simulink model "MVC2025_sim"  (R2024b)
settings: Solver=FixedStepAuto  StartTime=0.0  StopTime=Tsim  FixedStep=Ts
InitFcn:
  | warning('off','all')
StopFcn:
  | warning('on','all')
undefined symbols (not defined in the file or in its folder): BAT, BUS, CTRLpmsm, CTRLtug, CTRLves, DiscIntNeverNeededParam, ESM, GEN, magnitude, MOT, RLgain, SM, tau0, Ts, TUG, VES
libraries: fl_lib x47, nesl_utility x35, simulink x24, slpidlib x10, ee_lib x10, sdl_lib x3, rllib x1, batteryecm_lib x1
(part 3 of 3)

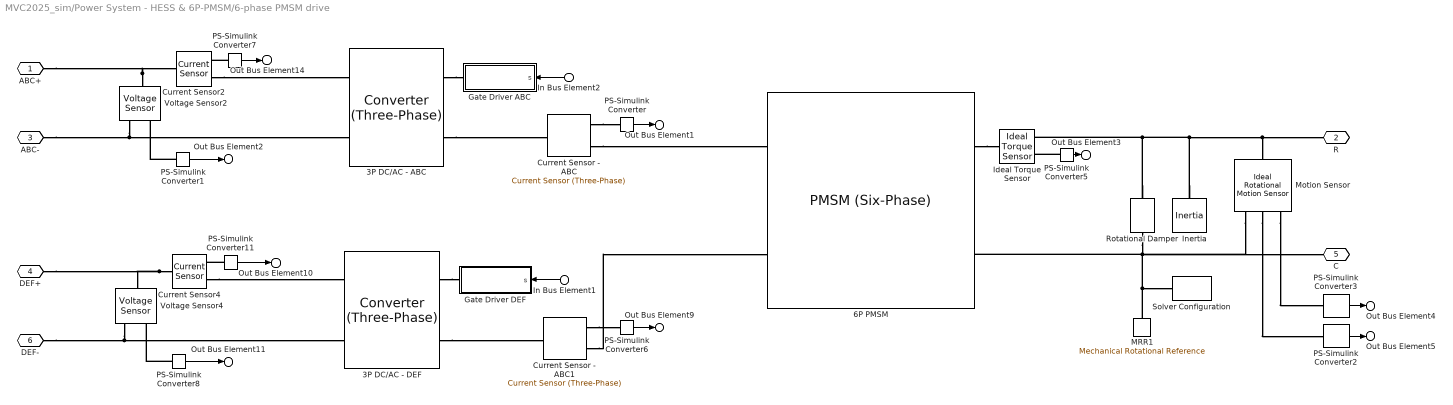
== system MVC2025_sim/Power System - HESS & 6P-PMSM/6-phase PMSM drive ==
  In Bus Element1 : Inport  PortName=CTRL  Element=SDEF
  In Bus Element2 : Inport  PortName=CTRL  Element=SABC
  3P DC/AC - ABC : ee_lib/Semiconductors & Converters/Converters/Converter (Three-Phase)  port_option=ee.enum.threePhasePort.composite  fidelity_option=ee.enum.converters.fidelity.detailed  device_type=ee.enum.converters.switchingdevice.averaged  showThermalPort=false  K=0  Vth=0.5 V  Vgt=1 V  Vgt_off=-1 V  Ih=1 A  Vf=0.01 V  Ron=0.001 Ohm  Rds=0.001 Ohm  Goff=1e-6 1/Ohm  Eon_scalar=22.86e-3 J  Eoff_scalar=17.14e-3 J  Eoff_natural_commutation=10e-3 J  Voff=300 V  Iout_scalar=600 A  onCurrentMeasDelay=0 s  useCurrentFromPreviousCycle=false  useVoltageFromPreviousCycle=false  diode_param=ee.enum.converters.protectiondiode.none  diode_Vf=0.01 V  diode_Ron=0.001 Ohm  diode_Goff=1e-5 1/Ohm  diode_C=50 nF  diode_iRM=-235 A  diode_iF=300 A  diode_idot=-50 A/us  diode_trr_param=ee.enum.converters.diodetrr.trr_factor  diode_trr_factor=3  diode_trr=15 us  diode_Qrr=1500 s*uA  diode_rec_loss_model=ee.enum.diode.reverseRecoveryModel.fixed  diode_ErecVal=0 J  diode_scaleWithIandV=false  diode_ErecMat=zeros(2, 3) J  diode_TjrecVec=[298.15, 398.15] K  diode_IfrecVec=[.1, 1, 10] A  diode_IrecVal=10 A  diode_VrecVal=10 V  diode_tFilter=1 / 1000 / 100 s  thermal_network_parameterization=ee.enum.thermalNetworkTopology.external  Rth=[.08, .5] K/W  Rth_Cauer=[.08, .1, .5] K/W  Rth_Foster=[.08, .14, .22, .16] K/W  thermal_mass_parameterization=ee.enum.thermalNetwork.timeconstant  thermal_mass=[.01, .5] J/K  thermal_mass_Cauer=[.01, .1, .5] J/K  thermal_mass_Foster=[.001, .005, .05, .5] J/K  thermal_time_constant=[.001, .2] s  thermal_time_constant_Cauer=[.001, .1, .2] s  thermal_time_constant_Foster=[7e-05, .0007, .01, .08] s  thermal_mass_initial_temperatures=[25, 25] degC  thermal_mass_initial_temperatures_Cauer=[25, 25, 25] degC  junction_thermal_mass=0.01 J/K  Tvec_initial_Foster=[25, 25, 25, 25] degC  snubber_type=ee.enum.converters.snubber.exclude  Cs=1e-7 F  Rs=0.1 Ohm  Vce_loss=[0, 150, 300] V
  3P DC/AC - DEF : ee_lib/Semiconductors & Converters/Converters/Converter (Three-Phase)  port_option=ee.enum.threePhasePort.composite  fidelity_option=ee.enum.converters.fidelity.detailed  device_type=ee.enum.converters.switchingdevice.averaged  showThermalPort=false  K=0  Vth=0.5 V  Vgt=1 V  Vgt_off=-1 V  Ih=1 A  Vf=0.01 V  Ron=0.001 Ohm  Rds=0.001 Ohm  Goff=1e-6 1/Ohm  Eon_scalar=22.86e-3 J  Eoff_scalar=17.14e-3 J  Eoff_natural_commutation=10e-3 J  Voff=300 V  Iout_scalar=600 A  onCurrentMeasDelay=0 s  useCurrentFromPreviousCycle=false  useVoltageFromPreviousCycle=false  diode_param=ee.enum.converters.protectiondiode.none  diode_Vf=0.01 V  diode_Ron=0.001 Ohm  diode_Goff=1e-5 1/Ohm  diode_C=50 nF  diode_iRM=-235 A  diode_iF=300 A  diode_idot=-50 A/us  diode_trr_param=ee.enum.converters.diodetrr.trr_factor  diode_trr_factor=3  diode_trr=15 us  diode_Qrr=1500 s*uA  diode_rec_loss_model=ee.enum.diode.reverseRecoveryModel.fixed  diode_ErecVal=0 J  diode_scaleWithIandV=false  diode_ErecMat=zeros(2, 3) J  diode_TjrecVec=[298.15, 398.15] K  diode_IfrecVec=[.1, 1, 10] A  diode_IrecVal=10 A  diode_VrecVal=10 V  diode_tFilter=1 / 1000 / 100 s  thermal_network_parameterization=ee.enum.thermalNetworkTopology.external  Rth=[.08, .5] K/W  Rth_Cauer=[.08, .1, .5] K/W  Rth_Foster=[.08, .14, .22, .16] K/W  thermal_mass_parameterization=ee.enum.thermalNetwork.timeconstant  thermal_mass=[.01, .5] J/K  thermal_mass_Cauer=[.01, .1, .5] J/K  thermal_mass_Foster=[.001, .005, .05, .5] J/K  thermal_time_constant=[.001, .2] s  thermal_time_constant_Cauer=[.001, .1, .2] s  thermal_time_constant_Foster=[7e-05, .0007, .01, .08] s  thermal_mass_initial_temperatures=[25, 25] degC  thermal_mass_initial_temperatures_Cauer=[25, 25, 25] degC  junction_thermal_mass=0.01 J/K  Tvec_initial_Foster=[25, 25, 25, 25] degC  snubber_type=ee.enum.converters.snubber.exclude  Cs=1e-7 F  Rs=0.1 Ohm  Vce_loss=[0, 150, 300] V
  6P PMSM : ee_lib/Electromechanical/Permanent Magnet/PMSM (Six-Phase)  nPolePairs=MOT.p  pmflux_param=ee.enum.pmflux.fluxlinkage  pm_flux_linkage=MOT.PMflux Wb  stator_param=ee.enum.statorparam.LdLqL0  Ld=MOT.Ls H  Lq=MOT.Ls H  L0=MOT.L0 H  Ls=0.0002 H  Lm=-0.00002 H  Ms=0.00002 H  Rs=MOT.R Ohm  zero_sequence=ee.enum.park.zerosequence.exclude  axes_param=ee.enum.rotorangle.daxis  torque_constant=0.18 N*m/A  back_emf_constant=0.18 V/(rad/s)  J=0.01*MOT.J kg*m^2  lam=0.01*MOT.D N*m/(rad/s)  i_ds_specify=on  i_ds_priority=High  i_ds=0 A  i_ds_nominal_specify=off  i_ds_nominal_value=1  i_ds_nominal_unit=A  i_qs_specify=on  i_qs_priority=High  i_qs=0 A  i_qs_nominal_specify=off  i_qs_nominal_value=1  i_qs_nominal_unit=A  i_z1_specify=on  i_z1_priority=High  i_z1=0 A  i_z1_nominal_specify=off  i_z1_nominal_value=1  i_z1_nominal_unit=A  i_z2_specify=on  i_z2_priority=High  i_z2=0 A  i_z2_nominal_specify=off  i_z2_nominal_value=1  i_z2_nominal_unit=A  torque_specify=on  torque_priority=High  torque=0 N*m  torque_nominal_specify=off  torque_nominal_value=1  torque_nominal_unit=N*m  angular_velocity_specify=on  angular_velocity_priority=High  angular_velocity=0 rpm  angular_velocity_nominal_specify=off  angular_velocity_nominal_value=1  angular_velocity_nominal_unit=rpm  angular_position_specify=on  angular_position_priority=High  angular_position=0 deg  angular_position_nominal_specify=off  angular_position_nominal_value=1  angular_position_nominal_unit=deg  Tmeas=298.15 K  alpha=3.93e-3 1/K  alpha_flux=-0.001 1/K  stator_thermal_mass=100 J/K  rotor_thermal_mass=200 J/K  temperatureA_specify=off  temperatureA_priority=High  temperatureA=25 degC  temperatureA_nominal_specify=off  temperatureA_nominal_value=1  temperatureA_nominal_unit=degC  temperatureB_specify=off  temperatureB_priority=High  temperatureB=25 degC  temperatureB_nominal_specify=off  temperatureB_nominal_value=1  temperatureB_nominal_unit=degC  temperatureC_specify=off  temperatureC_priority=High  temperatureC=25 degC  temperatureC_nominal_specify=off  temperatureC_nominal_value=1  temperatureC_nominal_unit=degC  temperatureX_specify=off  temperatureX_priority=High  temperatureX=25 degC  temperatureX_nominal_specify=off  temperatureX_nominal_value=1  temperatureX_nominal_unit=degC  temperatureY_specify=off  temperatureY_priority=High  temperatureY=25 degC  temperatureY_nominal_specify=off  temperatureY_nominal_value=1  temperatureY_nominal_unit=degC  temperatureZ_specify=off  temperatureZ_priority=High  temperatureZ=25 degC  temperatureZ_nominal_specify=off  temperatureZ_nominal_value=1  temperatureZ_nominal_unit=degC  temperatureR_specify=off  temperatureR_priority=High  temperatureR=25 degC  temperatureR_nominal_specify=off  temperatureR_nominal_value=1  temperatureR_nominal_unit=degC
      settings: InternalSimscapePortConfiguration="{\"Bottom\":[],\"Left\":[{\"id\":\"N1\",\"label\":\"~ABC\",\"type\":\"foundation.electrical.three_phase\"},{\"id\":\"N2\",\"label\":\"~XYZ\",\"type\":\"foundation.electrical.three_phase\"}],\"Right\":[{\"id\":\"R\",\"label\":\"R\",\"type\":\"foundation.mechanical.rotational.rotational\"},{\"id\":\"C\",\"label\":\"C\",\"type\":\"foundation.mechanical.rotational.rotational\"}],\"Top\":[]}"
  Current Sensor - ABC : ee_lib/Sensors & Transducers/Current Sensor (Three-Phase)
  Current Sensor - ABC1 : ee_lib/Sensors & Transducers/Current Sensor (Three-Phase)
  Current Sensor2 : fl_lib/Electrical/Electrical Sensors/Current Sensor
  Current Sensor4 : fl_lib/Electrical/Electrical Sensors/Current Sensor
  Gate Driver ABC : Subsystem
  Gate Driver DEF : Subsystem
  Ideal Torque Sensor : fl_lib/Mechanical/Mechanical Sensors/Ideal Torque Sensor
  Inertia : fl_lib/Mechanical/Rotational Elements/Inertia  inertia=0.99*MOT.J kg*m^2  num_ports=foundation.enum.numPorts2.one  w_specify=off  w_priority=High  w=0 rad/s  w_nominal_specify=off  w_nominal_value=1  w_nominal_unit=rad/s  t_specify=off  t_priority=None  t=0 N*m  t_nominal_specify=off  t_nominal_value=1  t_nominal_unit=N*m
  MRR1 : fl_lib/Mechanical/Rotational Elements/Mechanical Rotational Reference
  Motion Sensor : fl_lib/Mechanical/Mechanical Sensors/Ideal Rotational Motion Sensor  reference=foundation.enum.MeasurementReference.difference  acceleration_port=false  velocity_port=true  position_port=true  wrap_angle=simscape.enum.onoff.off  offset=0 rad
  PS-Simulink Converter{,6..7,11} (4 alike) : nesl_utility/PS-Simulink Converter  PhysicalDomain=network_engine_domain  SubClassName=ps_output  LeftPortType=input  RightPortType=output  PseudoPeriodic=off  Frequencies=[]  VectorFormat=1-D array  Unit=A  AffineConversion=off
  PS-Simulink Converter1 : nesl_utility/PS-Simulink Converter  PhysicalDomain=network_engine_domain  SubClassName=ps_output  LeftPortType=input  RightPortType=output  PseudoPeriodic=off  Frequencies=[]  VectorFormat=1-D array  Unit=V  AffineConversion=off
  PS-Simulink Converter2 : nesl_utility/PS-Simulink Converter  PhysicalDomain=network_engine_domain  SubClassName=ps_output  LeftPortType=input  RightPortType=output  PseudoPeriodic=off  Frequencies=[]  VectorFormat=1-D array  Unit=rad/s  AffineConversion=off
  PS-Simulink Converter3 : nesl_utility/PS-Simulink Converter  PhysicalDomain=network_engine_domain  SubClassName=ps_output  LeftPortType=input  RightPortType=output  PseudoPeriodic=off  Frequencies=[]  VectorFormat=1-D array  Unit=rad  AffineConversion=off
  PS-Simulink Converter5 : nesl_utility/PS-Simulink Converter  PhysicalDomain=network_engine_domain  SubClassName=ps_output  LeftPortType=input  RightPortType=output  PseudoPeriodic=off  Frequencies=[]  VectorFormat=1-D array  Unit=N*m  AffineConversion=off
  PS-Simulink Converter8 : nesl_utility/PS-Simulink Converter  PhysicalDomain=network_engine_domain  SubClassName=ps_output  LeftPortType=input  RightPortType=output  PseudoPeriodic=off  Frequencies=[]  VectorFormat=1-D array  Unit=V  AffineConversion=off
  Rotational Damper : fl_lib/Mechanical/Rotational Elements/Rotational Damper  D=0.99*MOT.D N*m/(rad/s)  w_specify=off  w_priority=None  w=0 rad/s  w_nominal_specify=off  w_nominal_value=1  w_nominal_unit=rad/s  t_specify=off  t_priority=None  t=0 N*m  t_nominal_specify=off  t_nominal_value=1  t_nominal_unit=N*m
  Solver Configuration : nesl_utility/Solver Configuration  PhysicalDomain=network_engine_domain  SubClassName=solver  LeftPortType=input  RightPortType=generic  Tones=[]  Harmonics=[]  SimulateNoise=off  Profile=off  UseLocalSampling=off  EnableSwitchedLinearOptims=on  FrequencyDomain=off  UseCCode=off  RelTol=0.001  AbsTol=1e-06  MinStep=1e-09  ToWorkspace=off  RevertToSquareIcSolve=off  NumHomotopyIterations=100  PhasorMode=off  PhasorModeNumHarmonics=1  ConsistencySolver=NEWTON_FTOL  IndexReductionMethod=DerivativeReplacement  DoDC=off  ResidualTolerance=1e-09  ConsistencyTolSource=GLOBAL  ConsistencyAbsTol=0.001  ConsistencyRelTol=0.001  ConsistencyTolFactor=0.001  UseLocalSolver=off  LocalSolverChoice=NE_PARTITIONING_ADVANCER  ResolveIndetEquations=on  FunctionEvalNumThread=1  LocalSolverSampleTime=1e-5  DoFixedCost=off  MaxNonlinIter=3  MaxModeIter=2  ComputeImpulses=off  ImpulseIterations=2  LinearAlgebra=auto  LinearAlgebraNumThread=0  EquationFormulation=NE_TIME_EF  DelaysMemoryBudget=1024  AutomaticFiltering=on  FilteringTimeConstant=0.001  PartitionStorageMethod=AS_NEEDED  PartitionMemoryBudget=1024  PartitionMethod=FAST  MultibodyUseLocalSolver=off  MultibodyLocalSolverChoice=ODE1  MultibodyLocalSolverSampleTime=0.001
  Voltage Sensor2 : fl_lib/Electrical/Electrical Sensors/Voltage Sensor
  Voltage Sensor4 : fl_lib/Electrical/Electrical Sensors/Voltage Sensor
  ABC+ : PMIOPort  Side=Left
  R : PMIOPort  Port=2  Side=Right
  ABC- : PMIOPort  Port=3  Side=Left
  DEF+ : PMIOPort  Port=4  Side=Left
  C : PMIOPort  Port=5  Side=Right
  DEF- : PMIOPort  Port=6  Side=Left
  Out Bus Element14 : Outport  PortName=DC  Element=iABC
  Out Bus Element10 : Outport  PortName=DC  Element=iDEF
  Out Bus Element11 : Outport  PortName=DC  Element=vDEF
  Out Bus Element2 : Outport  PortName=DC  Element=vABC
  Out Bus Element1 : Outport  Port=2  PortName=PMSM  Element=iABC
  Out Bus Element9 : Outport  Port=2  PortName=PMSM  Element=iDEF
  Out Bus Element3 : Outport  Port=2  PortName=PMSM  Element=Te
  Out Bus Element4 : Outport  Port=2  PortName=PMSM  Element=Om
  Out Bus Element5 : Outport  Port=2  PortName=PMSM  Element=wm
  wires:
  PS-Simulink Converter8/1 -> Out Bus Element11/1
  PS-Simulink Converter/1 -> Out Bus Element1/1
  PS-Simulink Converter6/1 -> Out Bus Element9/1
  PS-Simulink Converter7/1 -> Out Bus Element14/1
  PS-Simulink Converter1/1 -> Out Bus Element2/1
  In Bus Element1/1 -> Gate Driver DEF/1(s)
  PS-Simulink Converter11/1 -> Out Bus Element10/1
  In Bus Element2/1 -> Gate Driver ABC/1(s)
  PS-Simulink Converter5/1 -> Out Bus Element3/1
  PS-Simulink Converter2/1 -> Out Bus Element5/1
  PS-Simulink Converter3/1 -> Out Bus Element4/1
  connections:
  Current Sensor - ABC1/RConn1 -- PS-Simulink Converter6/LConn1
  3P DC/AC - ABC/LConn2 -- Current Sensor - ABC/LConn1
  Current Sensor2/RConn2 -- 3P DC/AC - ABC/RConn1
  Voltage Sensor2/LConn1 -- ABC+/RConn1 -- Current Sensor2/LConn1
  PS-Simulink Converter11/LConn1 -- Current Sensor4/RConn1
  Current Sensor - ABC/RConn1 -- PS-Simulink Converter/LConn1
  3P DC/AC - ABC/LConn1 -- Gate Driver ABC/RConn1
  Voltage Sensor2/RConn2 -- ABC-/RConn1 -- 3P DC/AC - ABC/RConn2
  3P DC/AC - DEF/LConn1 -- Gate Driver DEF/RConn1
  PS-Simulink Converter7/LConn1 -- Current Sensor2/RConn1
  PS-Simulink Converter8/LConn1 -- Voltage Sensor4/RConn1
  3P DC/AC - DEF/LConn2 -- Current Sensor - ABC1/LConn1
  Voltage Sensor4/RConn2 -- DEF-/RConn1 -- 3P DC/AC - DEF/RConn2
  Current Sensor4/LConn1 -- DEF+/RConn1 -- Voltage Sensor4/LConn1
  Current Sensor4/RConn2 -- 3P DC/AC - DEF/RConn1
  Current Sensor - ABC/RConn2 -- 6P PMSM/LConn1
  Current Sensor - ABC1/RConn2 -- 6P PMSM/LConn2
  PS-Simulink Converter1/LConn1 -- Voltage Sensor2/RConn1
  Inertia/LConn1 -- R/RConn1 -- Motion Sensor/LConn1 -- Ideal Torque Sensor/RConn1 -- Rotational Damper/LConn1
  MRR1/LConn1 -- Solver Configuration/RConn1 -- C/RConn1 -- Motion Sensor/RConn1 -- Rotational Damper/RConn1 -- 6P PMSM/RConn2
  Motion Sensor/RConn3 -- PS-Simulink Converter3/LConn1
  PS-Simulink Converter5/LConn1 -- Ideal Torque Sensor/RConn2
  Motion Sensor/RConn2 -- PS-Simulink Converter2/LConn1
  6P PMSM/RConn1 -- Ideal Torque Sensor/LConn1

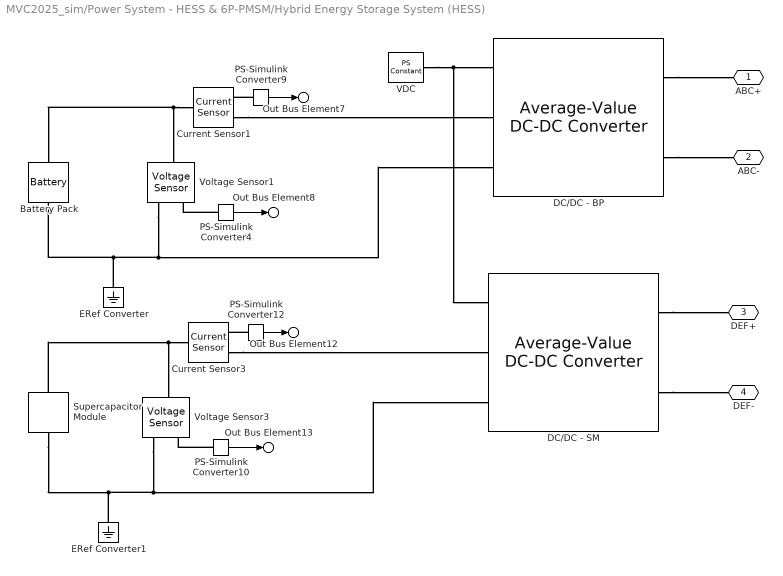
== system MVC2025_sim/Power System - HESS & 6P-PMSM/Hybrid Energy Storage System (HESS) ==
  Battery Pack : batteryecm_lib/Battery  Vnom=BAT.V_nom V  prm_dir=1  R1_dis=2 Ohm  R1_ch=2 Ohm  R1=BAT.r Ohm  prm_AH=2  AH=BAT.Q_nom C  V1=0.95*BAT.V_nom V  AH1=0.5*BAT.Q_nom C  prm_R2=1  R2=2000 Ohm  Tmeas=298.15 K  charge_measurement_port=simscape.enum.battery.enable.no  prm_dyn=2  Rp1=BAT.rho Ohm  tau1=BAT.rho*BAT.ci s  Rp2=0.005 Ohm  tau2=30 s  Rp3=0.005 Ohm  tau3=30 s  Rp4=0.005 Ohm  tau4=30 s  Rp5=0.005 Ohm  tau5=30 s  prm_fade=1  N_fade=100  AH_fade=45 A*hr  R1_fade=2.02 Ohm  R1_ch_fade=2.02 Ohm  V1_fade=10.35 V  prm_age=1  prm_age_OCV=1  OCV_age=0.9  SOC_age=60  Tmeas_age=298.15 K  delta_time_age_vec=[0] d  temperature_age_vec=[273] K  OCV_scaling_age=2.2134e6  OCV_offset_age=1.632e6  temp_exp_age=0.515833569 V  t_exp_age=0.75  Vnom_T2=12 V  R1_T2=2.2 Ohm  R1_T2_dis=2.2 Ohm  R1_T2_ch=2.2 Ohm  V1_T2=11.4 V  R2_T2=2200 Ohm  Rp1_T2=0.005 Ohm  tau1_T2=30 s  Rp2_T2=0.005 Ohm  tau2_T2=30 s  Rp3_T2=0.005 Ohm  tau3_T2=30 s  Rp4_T2=0.005 Ohm  tau4_T2=30 s  Rp5_T2=0.005 Ohm  tau5_T2=30 s  Tmeas2=273.15 K  thermal_port=simscape.enum.thermaleffects.omit  thermal_mass=30000 J/K  i_specify=off  i_priority=None  i=0 A  i_nominal_specify=off  i_nominal_value=1  i_nominal_unit=A  v_specify=off  v_priority=None  v=0 V  v_nominal_specify=off  v_nominal_value=1  v_nominal_unit=V  charge_specify=on  charge_priority=High  charge=BAT.SoC_0*BAT.Q_nom C  charge_nominal_specify=off  charge_nominal_value=1  charge_nominal_unit=A*hr  num_cycles_specify=off  num_cycles_priority=High  num_cycles=0  num_cycles_nominal_specify=off  num_cycles_nominal_value=1  num_cycles_nominal_unit=1  temperature_specify=off  temperature_priority=High  temperature=298.15 K  temperature_nominal_specify=off  temperature_nominal_value=1  temperature_nominal_unit=K
  Current Sensor1 : fl_lib/Electrical/Electrical Sensors/Current Sensor
  Current Sensor3 : fl_lib/Electrical/Electrical Sensors/Current Sensor
  DC/DC - BP : ee_lib/Semiconductors & Converters/Converters/Average-Value DC-DC Converter  control_option=ee.enum.converters.controlinput.voltage  converter_type=ee.enum.converters.dcdctype.buck  efficiency_option=ee.enum.converters.efficiency.tabulated  efficiency_fixed=100  i_vec=CONV.BATi A  efficiency_vec=CONV.BATeta
      settings: InternalSimscapePortConfiguration="{\"Bottom\":[],\"Left\":[{\"id\":\"Vref\",\"label\":\"Vref\",\"type\":\"input\"},{\"id\":\"p1\",\"label\":\"1+\",\"type\":\"foundation.electrical.electrical\"},{\"id\":\"n1\",\"label\":\"1-\",\"type\":\"foundation.electrical.electrical\"}],\"Right\":[{\"id\":\"p2\",\"label\":\"2+\",\"type\":\"foundation.electrical.electrical\"},{\"id\":\"n2\",\"label\":\"2-\",\"type\":\"foundation.electrical.electrical\"}],\"Top\":[]}"
  DC/DC - SM : ee_lib/Semiconductors & Converters/Converters/Average-Value DC-DC Converter  control_option=ee.enum.converters.controlinput.voltage  converter_type=ee.enum.converters.dcdctype.buck  efficiency_option=ee.enum.converters.efficiency.tabulated  efficiency_fixed=100  i_vec=CONV.SMi A  efficiency_vec=CONV.SMeta
      settings: InternalSimscapePortConfiguration="{\"Bottom\":[],\"Left\":[{\"id\":\"Vref\",\"label\":\"Vref\",\"type\":\"input\"},{\"id\":\"p1\",\"label\":\"1+\",\"type\":\"foundation.electrical.electrical\"},{\"id\":\"n1\",\"label\":\"1-\",\"type\":\"foundation.electrical.electrical\"}],\"Right\":[{\"id\":\"p2\",\"label\":\"2+\",\"type\":\"foundation.electrical.electrical\"},{\"id\":\"n2\",\"label\":\"2-\",\"type\":\"foundation.electrical.electrical\"}],\"Top\":[]}"
  ERef Converter : fl_lib/Electrical/Electrical Elements/Electrical Reference
  ERef Converter1 : fl_lib/Electrical/Electrical Elements/Electrical Reference
  PS-Simulink Converter10 : nesl_utility/PS-Simulink Converter  PhysicalDomain=network_engine_domain  SubClassName=ps_output  LeftPortType=input  RightPortType=output  PseudoPeriodic=off  Frequencies=[]  VectorFormat=1-D array  Unit=V  AffineConversion=off
  PS-Simulink Converter12 : nesl_utility/PS-Simulink Converter  PhysicalDomain=network_engine_domain  SubClassName=ps_output  LeftPortType=input  RightPortType=output  PseudoPeriodic=off  Frequencies=[]  VectorFormat=1-D array  Unit=A  AffineConversion=off
  PS-Simulink Converter4 : nesl_utility/PS-Simulink Converter  PhysicalDomain=network_engine_domain  SubClassName=ps_output  LeftPortType=input  RightPortType=output  PseudoPeriodic=off  Frequencies=[]  VectorFormat=1-D array  Unit=V  AffineConversion=off
  PS-Simulink Converter9 : nesl_utility/PS-Simulink Converter  PhysicalDomain=network_engine_domain  SubClassName=ps_output  LeftPortType=input  RightPortType=output  PseudoPeriodic=off  Frequencies=[]  VectorFormat=1-D array  Unit=A  AffineConversion=off
  Supercapacitor Module : ee_lib/Passive/Supercapacitor  R=[SM.r, SM.rho_1, SM.rho_2] Ohm  C=[SM.C, SM.ci_1, SM.ci_2] F  Kv=SM.k F/V  R_discharge=inf Ohm  N_series=1  N_parallel=1  i_specify=off  i_priority=None  i=0 A  i_nominal_specify=off  i_nominal_value=1  i_nominal_unit=A  v_specify=off  v_priority=High  v=VSM_0 V  v_nominal_specify=off  v_nominal_value=1  v_nominal_unit=V  vc1_specify=on  vc1_priority=High  vc1=SM.V_0 V  vc1_nominal_specify=off  vc1_nominal_value=1  vc1_nominal_unit=V  vc2_specify=on  vc2_priority=High  vc2=SM.V_0 V  vc2_nominal_specify=off  vc2_nominal_value=1  vc2_nominal_unit=V  vc3_specify=off  vc3_priority=High  vc3=VSM_0 V  vc3_nominal_specify=off  vc3_nominal_value=1  vc3_nominal_unit=V
      settings: InternalSimscapePortConfiguration="{\"Bottom\":[],\"Left\":[{\"id\":\"p\",\"label\":\"+\",\"type\":\"foundation.electrical.electrical\"}],\"Right\":[{\"id\":\"n\",\"label\":\"-\",\"type\":\"foundation.electrical.electrical\"}],\"Top\":[]}"
  VDC : fl_lib/Physical Signals/Sources/PS Constant  constant=BUS.Vdc V
  Voltage Sensor1 : fl_lib/Electrical/Electrical Sensors/Voltage Sensor
  Voltage Sensor3 : fl_lib/Electrical/Electrical Sensors/Voltage Sensor
  ABC+ : PMIOPort  Side=Right
  ABC- : PMIOPort  Port=2  Side=Right
  DEF+ : PMIOPort  Port=3  Side=Right
  DEF- : PMIOPort  Port=4  Side=Right
  Out Bus Element7 : Outport  PortName=HESS  Element=iBP
  Out Bus Element8 : Outport  PortName=HESS  Element=vBP
  Out Bus Element12 : Outport  PortName=HESS  Element=iSM
  Out Bus Element13 : Outport  PortName=HESS  Element=vSM
  wires:
  PS-Simulink Converter4/1 -> Out Bus Element8/1
  PS-Simulink Converter9/1 -> Out Bus Element7/1
  PS-Simulink Converter10/1 -> Out Bus Element13/1
  PS-Simulink Converter12/1 -> Out Bus Element12/1
  connections:
  Current Sensor1/RConn2 -- DC/DC - BP/LConn2
  Voltage Sensor1/RConn2 -- DC/DC - BP/LConn3 -- Battery Pack/RConn1 -- ERef Converter/LConn1
  VDC/RConn1 -- DC/DC - SM/LConn1 -- DC/DC - BP/LConn1
  PS-Simulink Converter4/LConn1 -- Voltage Sensor1/RConn1
  Current Sensor3/RConn2 -- DC/DC - SM/LConn2
  Current Sensor1/LConn1 -- Battery Pack/LConn1 -- Voltage Sensor1/LConn1
  Supercapacitor Module/RConn1 -- Voltage Sensor3/RConn2 -- DC/DC - SM/LConn3 -- ERef Converter1/LConn1
  PS-Simulink Converter9/LConn1 -- Current Sensor1/RConn1
  Supercapacitor Module/LConn1 -- Current Sensor3/LConn1 -- Voltage Sensor3/LConn1
  DC/DC - BP/RConn2 -- ABC-/RConn1
  PS-Simulink Converter12/LConn1 -- Current Sensor3/RConn1
  PS-Simulink Converter10/LConn1 -- Voltage Sensor3/RConn1
  DC/DC - SM/RConn1 -- DEF+/RConn1
  DC/DC - BP/RConn1 -- ABC+/RConn1
  DC/DC - SM/RConn2 -- DEF-/RConn1

== system MVC2025_sim/Propeller - Tug + Vessel/Tug + Ves Resistance ==
  ...2 : fl_lib/Physical Signals/Functions/PS Gain  gain=0.5
  Operating mode : simulink/Sources/Repeating Sequence  rep_seq_t=V_star.time  rep_seq_y=V_star.mode
  PS Add : fl_lib/Physical Signals/Functions/PS Add
  PS Product2 : fl_lib/Physical Signals/Functions/PS Product
  Simulink-PS Converter : nesl_utility/Simulink-PS Converter  PhysicalDomain=network_engine_domain  SubClassName=ps_input  LeftPortType=input  RightPortType=output  PseudoPeriodic=off  Frequencies=[]  NoiseDistribution=none  NoiseParameters=[]  Unit=1  AffineConversion=off  FilteringAndDerivatives=provide  SimscapeFilterOrder=1  InputFilterTimeConstant=0.001  UdotUserProvided=0
  Tug Resistance : Subsystem
  Vessel Resistance : Subsystem
  vs : PMIOPort  Side=Left
  vw : PMIOPort  Port=2  Side=Left
  Fr : PMIOPort  Port=3  Side=Right
  wires:
  Operating mode/1 -> Simulink-PS Converter/1
  connections:
  ...2/RConn1 -- Fr/RConn1
  Vessel Resistance/LConn2 -- Tug Resistance/LConn2 -- vw/RConn1
  Vessel Resistance/RConn1 -- PS Product2/LConn1
  PS Add/RConn1 -- ...2/LConn1
  Tug Resistance/RConn1 -- PS Add/LConn1
  Vessel Resistance/LConn1 -- vs/RConn1 -- Tug Resistance/LConn1
  Simulink-PS Converter/RConn1 -- PS Product2/LConn2
  PS Product2/RConn1 -- PS Add/LConn2

== system MVC2025_sim/Power System - HESS & 6P-PMSM/6-phase PMSM drive/Gate Driver ABC ==
  s : Inport
  Demux : Demux  Outputs=6
  Simulink-PS Converter{1..6} (6 alike) : nesl_utility/Simulink-PS Converter  PhysicalDomain=network_engine_domain  SubClassName=ps_input  LeftPortType=input  RightPortType=output  PseudoPeriodic=off  Frequencies=[]  NoiseDistribution=none  NoiseParameters=[]  Unit=1  AffineConversion=off  FilteringAndDerivatives=zero  SimscapeFilterOrder=1  InputFilterTimeConstant=0.001  UdotUserProvided=1
  Six-Pulse Gate Multiplexer : ee_lib/Semiconductors & Converters/Converters/Six-Pulse Gate Multiplexer  port_option=ee.enum.controlport.ps
  g : PMIOPort  Side=Right
  wires:
  s/1 -> Demux/1
  Demux/1 -> Simulink-PS Converter1/1
  Demux/2 -> Simulink-PS Converter2/1
  Demux/5 -> Simulink-PS Converter5/1
  Demux/6 -> Simulink-PS Converter6/1
  Demux/3 -> Simulink-PS Converter3/1
  Demux/4 -> Simulink-PS Converter4/1
  connections:
  Six-Pulse Gate Multiplexer/LConn5 -- Simulink-PS Converter5/RConn1
  Six-Pulse Gate Multiplexer/LConn2 -- Simulink-PS Converter2/RConn1
  Simulink-PS Converter6/RConn1 -- Six-Pulse Gate Multiplexer/LConn6
  Six-Pulse Gate Multiplexer/RConn1 -- g/RConn1
  Six-Pulse Gate Multiplexer/LConn3 -- Simulink-PS Converter3/RConn1
  Six-Pulse Gate Multiplexer/LConn1 -- Simulink-PS Converter1/RConn1
  Six-Pulse Gate Multiplexer/LConn4 -- Simulink-PS Converter4/RConn1

== system MVC2025_sim/Power System - HESS & 6P-PMSM/6-phase PMSM drive/Gate Driver DEF ==
  s : Inport
  Demux : Demux  Outputs=6
  Simulink-PS Converter{1..6} (6 alike) : nesl_utility/Simulink-PS Converter  PhysicalDomain=network_engine_domain  SubClassName=ps_input  LeftPortType=input  RightPortType=output  PseudoPeriodic=off  Frequencies=[]  NoiseDistribution=none  NoiseParameters=[]  Unit=1  AffineConversion=off  FilteringAndDerivatives=zero  SimscapeFilterOrder=1  InputFilterTimeConstant=0.001  UdotUserProvided=1
  Six-Pulse Gate Multiplexer : ee_lib/Semiconductors & Converters/Converters/Six-Pulse Gate Multiplexer  port_option=ee.enum.controlport.ps
  g : PMIOPort  Side=Right
  wires:
  Demux/4 -> Simulink-PS Converter4/1
  Demux/3 -> Simulink-PS Converter3/1
  Demux/6 -> Simulink-PS Converter6/1
  Demux/5 -> Simulink-PS Converter5/1
  Demux/2 -> Simulink-PS Converter2/1
  Demux/1 -> Simulink-PS Converter1/1
  s/1 -> Demux/1
  connections:
  Six-Pulse Gate Multiplexer/LConn4 -- Simulink-PS Converter4/RConn1
  Six-Pulse Gate Multiplexer/LConn1 -- Simulink-PS Converter1/RConn1
  Six-Pulse Gate Multiplexer/LConn3 -- Simulink-PS Converter3/RConn1
  Six-Pulse Gate Multiplexer/RConn1 -- g/RConn1
  Simulink-PS Converter6/RConn1 -- Six-Pulse Gate Multiplexer/LConn6
  Six-Pulse Gate Multiplexer/LConn2 -- Simulink-PS Converter2/RConn1
  Six-Pulse Gate Multiplexer/LConn5 -- Simulink-PS Converter5/RConn1

== system MVC2025_sim/Propeller - Tug + Vessel/Tug + Ves Resistance/Tug Resistance ==
  ... : fl_lib/Physical Signals/Functions/PS Gain  gain=0.5*GEN.rhow*TUG.S kg/m
  Froude's num : fl_lib/Physical Signals/Functions/PS Gain  gain=1/sqrt(GEN.g*TUG.L) s/m
  PS Product : fl_lib/Physical Signals/Functions/PS Product
  PS Product1 : fl_lib/Physical Signals/Functions/PS Product
  PS Sign : fl_lib/Physical Signals/Nonlinear Operators/PS Sign
      settings: InternalSimscapePortConfiguration="{\"Bottom\":[],\"Left\":[{\"id\":\"I\",\"label\":\"\",\"type\":\"input\"}],\"Right\":[{\"id\":\"O\",\"label\":\"\",\"type\":\"output\"}],\"Top\":[]}"
  V^2 : fl_lib/Physical Signals/Functions/PS Math Function  fcn_choice=foundation.enum.math_function.square  v=1
  f : fl_lib/Physical Signals/Lookup Tables/PS Lookup Table (1D)  x=[0.05 0.2 0.3 0.4 0.5 0.6]  f=[0.003 0.0035 0.004 0.005 0.007 0.0065]  interp_method=simscape.enum.interpolation.smooth  extrap_method=simscape.enum.extrapolation.nearest
  rel speed : fl_lib/Physical Signals/Functions/PS Subtract
  vs : PMIOPort  Side=Left
  vw : PMIOPort  Port=2  Side=Left
  Fres : PMIOPort  Port=3  Side=Right
  connections:
  .../LConn1 -- PS Product/RConn1
  f/RConn1 -- PS Product/LConn2
  Froude's num/RConn1 -- f/LConn1
  V^2/RConn1 -- PS Product/LConn1
  PS Sign/RConn1 -- PS Product1/LConn1
  .../RConn1 -- PS Product1/LConn2
  PS Product1/RConn1 -- Fres/RConn1
  rel speed/LConn2 -- vw/RConn1
  rel speed/RConn1 -- V^2/LConn1 -- PS Sign/LConn1 -- Froude's num/LConn1
  vs/RConn1 -- rel speed/LConn1

== system MVC2025_sim/Propeller - Tug + Vessel/Tug + Ves Resistance/Vessel Resistance ==
  ... : fl_lib/Physical Signals/Functions/PS Gain  gain=0.5*GEN.rhow*VES.S kg/m
  Froude's num : fl_lib/Physical Signals/Functions/PS Gain  gain=1/sqrt(GEN.g*VES.L) s/m
  PS Product : fl_lib/Physical Signals/Functions/PS Product
  PS Product1 : fl_lib/Physical Signals/Functions/PS Product
  PS Sign : fl_lib/Physical Signals/Nonlinear Operators/PS Sign
      settings: InternalSimscapePortConfiguration="{\"Bottom\":[],\"Left\":[{\"id\":\"I\",\"label\":\"\",\"type\":\"input\"}],\"Right\":[{\"id\":\"O\",\"label\":\"\",\"type\":\"output\"}],\"Top\":[]}"
  V^2 : fl_lib/Physical Signals/Functions/PS Math Function  fcn_choice=foundation.enum.math_function.square  v=1
  f : fl_lib/Physical Signals/Lookup Tables/PS Lookup Table (1D)  x=[0.05 0.2 0.3 0.4 0.5 0.6]  f=[0.003 0.0035 0.004 0.005 0.007 0.0065]  interp_method=simscape.enum.interpolation.smooth  extrap_method=simscape.enum.extrapolation.nearest
  rel speed : fl_lib/Physical Signals/Functions/PS Subtract
  vs : PMIOPort  Side=Left
  vw : PMIOPort  Port=2  Side=Left
  Fres : PMIOPort  Port=3  Side=Right
  connections:
  vs/RConn1 -- rel speed/LConn1
  Froude's num/LConn1 -- PS Sign/LConn1 -- V^2/LConn1 -- rel speed/RConn1
  rel speed/LConn2 -- vw/RConn1
  Fres/RConn1 -- PS Product1/RConn1
  .../RConn1 -- PS Product1/LConn2
  PS Sign/RConn1 -- PS Product1/LConn1
  V^2/RConn1 -- PS Product/LConn1
  Froude's num/RConn1 -- f/LConn1
  f/RConn1 -- PS Product/LConn2
  .../LConn1 -- PS Product/RConn1
